simulink model "sampleModel1426_2_sub_sub_sub"  (R2023a)
settings: Solver=VariableStepAuto  StartTime=0.0  StopTime=10.0  RelTol=1e-3
libraries: hdlsllib x6, simulink x3
settings Model: Creator=user1  LastModifiedBy=user1
settings OptimizationCC: BlockReduction=off  ConditionallyExecuteInputs=off

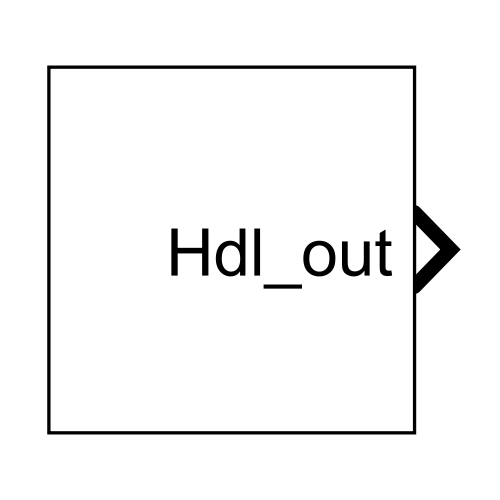
[thumbnail: Simulink's stored preview of the top-level diagram]
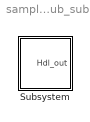
== system sampleModel1426_2_sub_sub_sub ==
  Subsystem : Subsystem

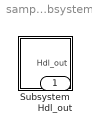
== system sampleModel1426_2_sub_sub_sub/Subsystem ==
  Subsystem : Subsystem
  Hdl_out : Outport  OutDataTypeStr=uint8

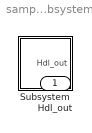
== system sampleModel1426_2_sub_sub_sub/Subsystem/Subsystem ==
  Subsystem : Subsystem
  Hdl_out : Outport  OutDataTypeStr=uint8

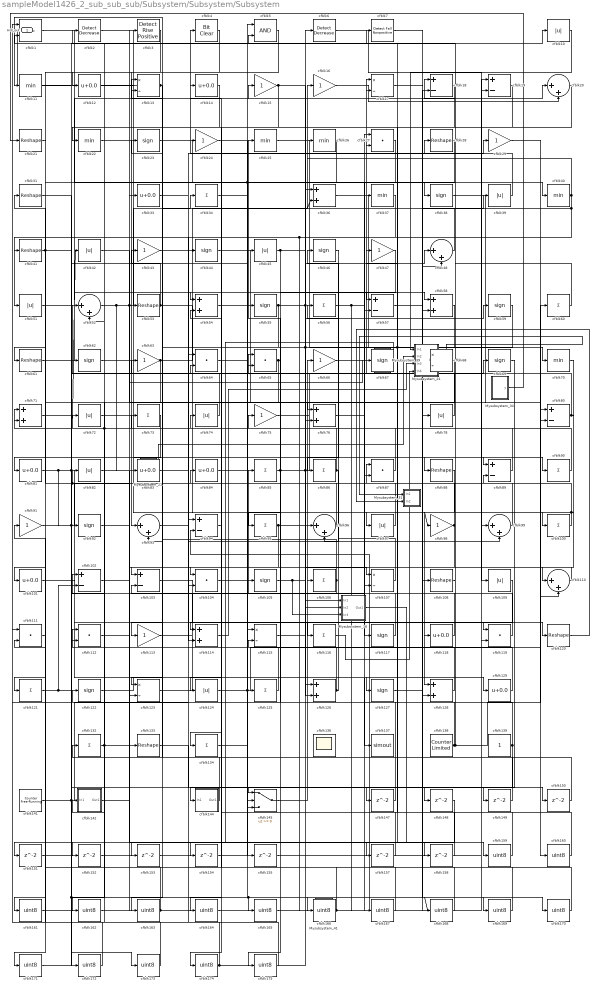
== system sampleModel1426_2_sub_sub_sub/Subsystem/Subsystem/Subsystem ==
  Mysubsystem_16 : Subsystem  TreatAsAtomicUnit=on  RTWFcnName=Mysubsystem_16
      settings: RTWFcnNameOpts=User specified  RTWFileNameOpts=Use function name
  Mysubsystem_21 : Subsystem  TreatAsAtomicUnit=on  RTWFcnName=Mysubsystem_21
      settings: RTWFcnNameOpts=User specified  RTWFileNameOpts=Use function name
  Mysubsystem_24 : Subsystem  TreatAsAtomicUnit=on  RTWFcnName=Mysubsystem_24
      settings: RTWFcnNameOpts=User specified  RTWFileNameOpts=Use function name
  Mysubsystem_31 : Subsystem  TreatAsAtomicUnit=on  RTWFcnName=Mysubsystem_31
      settings: RTWFcnNameOpts=User specified  RTWFileNameOpts=Use function name
  Mysubsystem_34 : Subsystem  TreatAsAtomicUnit=on  RTWFcnName=Mysubsystem_34
      settings: RTWFcnNameOpts=User specified  RTWFileNameOpts=Use function name
  Mysubsystem_39 : Subsystem  TreatAsAtomicUnit=on  RTWFcnName=Mysubsystem_39
      settings: RTWFcnNameOpts=User specified  RTWFileNameOpts=Use function name
  Mysubsystem_41 : Subsystem  TreatAsAtomicUnit=on  RTWFcnName=Mysubsystem_41
      settings: RTWFcnNameOpts=User specified  RTWFileNameOpts=Use function name
  cfblk1 : RelationalOperator  Operator=<=  OutDataTypeStr=boolean  InputSameDT=off
  cfblk{10,39,42,45,51,72,74,78,82,97,109,124} (12 alike) : Abs  OutDataTypeStr=uint8  SaturateOnIntegerOverflow=off
  cfblk{34,56,60,73,85..86,90,95,100,106,116,121,125,132,134} (15 alike) : Sum  Inputs=+  OutDataTypeStr=uint8
  cfblk{12,14,33,81,83..84,101,118,129} (9 alike) : Bias  Bias=0.0  SaturateOnIntegerOverflow=off
  cfblk{18..19,57,80,89,94,102..103} (8 alike) : Sum  Inputs=+-  OutDataTypeStr=uint8
  cfblk{27,64..65,87,104,111..112,119} (8 alike) : DotProduct  OutDataTypeStr=uint8
  cfblk{23,38,44,46,55,59,62,67,69,92,105,117,122,127} (14 alike) : Signum
  cfblk{13,17,68,107,115,123} (6 alike) : Product  Inputs=*/  OutDataTypeStr=uint8  RndMeth=Zero  SaturateOnIntegerOverflow=on
  cfblk{21,28,31,41,53,61,88,108,120,133} (10 alike) : Reshape
  cfblk{11,22,25..26,37,40,70} (7 alike) : MinMax  OutDataTypeStr=uint8
  cfblk{20,48,52,93,96,99,110} (7 alike) : Sum  Inputs=|++  OutDataTypeStr=uint8
  cfblk{15..16,24,29,43,47,63,66,75,91,98,113} (12 alike) : Gain  OutDataTypeStr=uint8
  cfblk{36,54,58,71,76,114,126,128} (8 alike) : Sum  OutDataTypeStr=uint8
  cfblk136 : Scope
      settings: Floating=on
  cfblk137 : ToWorkspace  VariableName=simout  SaveFormat=Timeseries  SampleTime=-1
  cfblk138 : hdlsllib/Sources/Counter Limited  uplimit=7  tsamp=-1
  cfblk139 : Constant  OutDataTypeStr=uint8  SampleTime=-1
  cfblk141 : hdlsllib/Sources/Counter Free-Running  NumBits=16  tsamp=-1
  cfblk142 : Subsystem
      settings: LibrarySourceBlock=|
      | hdlsllib/Ports &
      | Subsystems/Subsystem
  cfblk144 : Subsystem
      settings: LibrarySourceBlock=|
      | hdlsllib/Ports &
      | Subsystems/Subsystem
  cfblk145 : Switch  OutDataTypeStr=uint8  SaturateOnIntegerOverflow=off  InputSameDT=off
  cfblk{147..155,157..158} (11 alike) : Delay  SampleTime=1
  cfblk{159..175} (17 alike) : DataTypeConversion  OutDataTypeStr=uint8  SaturateOnIntegerOverflow=off  RndMeth=Floor
  cfblk2 : simulink/Logic and Bit Operations/Detect Decrease  vinit=0.0  OutDataTypeStr=uint8
      settings: LibrarySourceBlock=|
      | hdlsllib/Logic and Bit
      | Operations/Detect
      | Decrease
  cfblk3 : hdlsllib/Logic and Bit Operations/Detect Rise Positive  vinit=0  OutDataTypeStr=uint8
  cfblk4 : simulink/Logic and Bit Operations/Bit Clear  iBit=0
      settings: LibrarySourceBlock=|
      | hdlsllib/Logic and Bit
      | Operations/Bit Clear
  cfblk5 : Logic  AllPortsSameDT=off  OutDataTypeStr=boolean
  cfblk6 : simulink/Logic and Bit Operations/Detect Decrease  vinit=0.0  OutDataTypeStr=uint8
      settings: LibrarySourceBlock=|
      | hdlsllib/Logic and Bit
      | Operations/Detect
      | Decrease
  cfblk7 : hdlsllib/Logic and Bit Operations/Detect Fall Nonpositive  vinit=0  OutDataTypeStr=uint8
  Hdl_out : Outport  OutDataTypeStr=uint8
  wires:
  cfblk2/1 -> cfblk88/1
  cfblk48/1 -> cfblk11/1
  cfblk5/1 -> cfblk93/1
  cfblk54/1 -> cfblk25/1
  cfblk52/1 -> cfblk83/1, cfblk80/2, cfblk34/1
  cfblk64/1 -> cfblk166/1
  cfblk119/1 -> cfblk85/1
  cfblk117/1 -> cfblk66/1
  cfblk108/1 -> cfblk18/1
  cfblk53/1 -> cfblk43/1, cfblk97/1
  cfblk75/1 -> cfblk17/1
  cfblk33/1 -> cfblk29/1
  cfblk62/1 -> cfblk90/1
  cfblk61/1 -> cfblk15/1
  cfblk68/1 -> cfblk113/1
  cfblk101/1 -> cfblk120/1
  cfblk94/1 -> cfblk174/1
  cfblk1/1 -> cfblk38/1
  cfblk88/1 -> cfblk128/1
  cfblk56/1 -> cfblk167/1, cfblk117/1
  cfblk145/1 -> cfblk106/1
  cfblk58/1 -> cfblk157/1, cfblk123/1
  cfblk124/1 -> cfblk17/2, cfblk60/1
  cfblk6/1 -> cfblk99/1
  cfblk45/1 -> cfblk175/1, cfblk28/1
  cfblk110/1 -> cfblk104/1
  cfblk80/1 -> cfblk13/2, cfblk110/1
  cfblk38/1 -> cfblk110/2
  cfblk82/1 -> cfblk133/1
  cfblk122/1 -> cfblk127/1
  cfblk63/1 -> cfblk121/1, cfblk16/1
  cfblk107/1 -> cfblk75/1
  cfblk20/1 -> cfblk128/2
  cfblk72/1 -> cfblk118/1
  cfblk25/1 -> cfblk108/1
  cfblk74/1 -> cfblk63/1
  cfblk73/1 -> cfblk81/1
  cfblk12/1 -> cfblk40/1
  cfblk89/1 -> cfblk2/1, cfblk42/1
  cfblk36/1 -> cfblk70/1
  cfblk127/1 -> cfblk39/1
  cfblk141/1 -> cfblk44/1, cfblk173/1, cfblk168/1, cfblk165/1
  cfblk100/1 -> cfblk89/2, cfblk98/1
  cfblk85/1 -> cfblk65/1, cfblk59/1, cfblk69/1
  cfblk132/1 -> cfblk112/1, cfblk67/1
  cfblk86/1 -> cfblk96/2, cfblk71/1
  cfblk123/1 -> cfblk6/1
  cfblk103/1 -> cfblk116/1
  cfblk43/1 -> cfblk76/1
  cfblk144/1(Out1) -> cfblk132/1
  cfblk4/1 -> cfblk12/1
  cfblk129/1 -> cfblk115/2
  cfblk11/1 -> cfblk5/2
  cfblk118/1 -> cfblk87/1
  cfblk142/1(Out1) -> cfblk53/1
  cfblk22/1 -> cfblk57/1
  cfblk81/1 -> cfblk92/1, cfblk10/1, cfblk137/1
  cfblk44/1 -> cfblk109/1
  cfblk125/1 -> cfblk73/1
  cfblk83/1 -> cfblk99/2
  cfblk66/1 -> cfblk119/1
  cfblk90/1 -> cfblk23/1
  cfblk37/1 -> cfblk51/1
  cfblk21/1 -> cfblk61/1
  cfblk113/1 -> cfblk37/1
  cfblk39/1 -> cfblk4/1
  cfblk92/1 -> cfblk20/1
  cfblk93/1 -> cfblk27/2
  cfblk34/1 -> cfblk129/1
  cfblk51/1 -> cfblk54/1
  cfblk106/1 -> cfblk103/2, cfblk72/1
  cfblk26/1 -> cfblk114/1
  cfblk138/1 -> cfblk55/1, cfblk80/1, cfblk68/1
  cfblk121/1 -> cfblk102/2, cfblk105/1
  cfblk14/1 -> cfblk22/1
  cfblk19/1 -> cfblk163/1
  cfblk104/1 -> cfblk125/1
  cfblk139/1 -> cfblk52/2, cfblk144/1(In1)
  cfblk96/1 -> cfblk56/1, cfblk71/2, cfblk82/1
  cfblk46/1 -> cfblk86/1
  cfblk128/1 -> cfblk54/2
  cfblk41/1 -> cfblk145/3, cfblk101/1
  cfblk95/1 -> cfblk123/2, cfblk36/1
  cfblk115/1 -> cfblk48/1
  cfblk59/1 -> cfblk134/1, Mysubsystem_16/2(In2)
  cfblk16/1 -> cfblk20/2
  cfblk126/1 -> cfblk102/1, cfblk46/1
  cfblk70/1 -> cfblk100/1
  cfblk109/1 -> cfblk124/1
  cfblk87/1 -> cfblk74/1
  cfblk15/1 -> cfblk164/1, cfblk107/2
  cfblk55/1 -> cfblk103/1, cfblk58/1, Mysubsystem_16/1(In1)
  cfblk78/1 -> cfblk52/1
  cfblk105/1 -> cfblk107/1, Mysubsystem_16/3(In3)
  cfblk98/1 -> cfblk13/1, cfblk104/2
  cfblk28/1 -> cfblk57/2
  cfblk91/1 -> cfblk45/1, cfblk33/1
  cfblk60/1 -> cfblk1/2
  cfblk47/1 -> cfblk145/1
  cfblk23/1 -> cfblk126/2
  cfblk97/1 -> cfblk31/1
  cfblk27/1 -> cfblk65/2, cfblk41/1
  cfblk57/1 -> cfblk18/2
  cfblk40/1 -> cfblk26/1, cfblk36/2, cfblk114/2, Mysubsystem_41/1(In1)
  cfblk71/1 -> cfblk68/2
  cfblk67/1 -> cfblk47/1
  cfblk99/1 -> cfblk24/1
  cfblk65/1 -> cfblk152/1, cfblk95/1
  cfblk76/1 -> cfblk89/1
  cfblk18/1 -> cfblk147/1
  cfblk147/1 -> cfblk1/1
  cfblk133/1 -> cfblk148/1
  cfblk69/1 -> cfblk149/1
  cfblk149/1 -> cfblk93/2
  cfblk134/1 -> cfblk150/1
  cfblk150/1 -> cfblk126/1
  cfblk151/1 -> cfblk119/2
  cfblk152/1 -> cfblk145/2
  cfblk13/1 -> Hdl_out/1, cfblk153/1
  cfblk153/1 -> cfblk96/1
  cfblk154/1 -> cfblk48/2
  cfblk24/1 -> cfblk155/1
  cfblk155/1 -> cfblk27/1
  cfblk157/1 -> cfblk115/1
  cfblk102/1 -> cfblk158/1
  cfblk158/1 -> cfblk5/1
  cfblk7/1 -> cfblk159/1
  cfblk159/1 -> cfblk14/1
  cfblk29/1 -> cfblk160/1
  cfblk160/1 -> cfblk7/1
  cfblk3/1 -> cfblk161/1
  cfblk161/1 -> cfblk78/1
  cfblk148/1 -> cfblk162/1
  cfblk162/1 -> cfblk3/1
  cfblk163/1 -> cfblk87/2, cfblk112/2
  cfblk164/1 -> cfblk19/1
  cfblk165/1 -> cfblk19/2
  cfblk166/1 -> cfblk91/1, cfblk58/2
  cfblk167/1 -> cfblk64/1
  cfblk168/1 -> cfblk64/2
  cfblk84/1 -> cfblk169/1
  cfblk169/1 -> cfblk142/1(In1)
  cfblk17/1 -> cfblk170/1
  cfblk170/1 -> cfblk84/1
  cfblk111/1 -> cfblk171/1
  cfblk171/1 -> cfblk62/1
  cfblk31/1 -> cfblk172/1
  cfblk172/1 -> cfblk111/1
  cfblk173/1 -> cfblk111/2
  cfblk174/1 -> cfblk122/1, cfblk76/2
  cfblk175/1 -> cfblk94/1
  Mysubsystem_16/1(Out1) -> cfblk151/1
  cfblk112/1 -> Mysubsystem_21/1(In1)
  cfblk10/1 -> Mysubsystem_24/1(In1)
  Mysubsystem_21/1(Out1) -> Mysubsystem_24/2(In2)
  cfblk114/1 -> Mysubsystem_24/3(In3)
  cfblk116/1 -> Mysubsystem_24/4(In4)
  Mysubsystem_24/1(Out1) -> Mysubsystem_31/1(In1)
  cfblk120/1 -> Mysubsystem_31/2(In2)
  Mysubsystem_34/1(y) -> cfblk21/1
  cfblk42/1 -> Mysubsystem_39/1(In1)
  Mysubsystem_39/1(Out1) -> cfblk154/1
  Mysubsystem_41/1(Out1) -> cfblk94/2

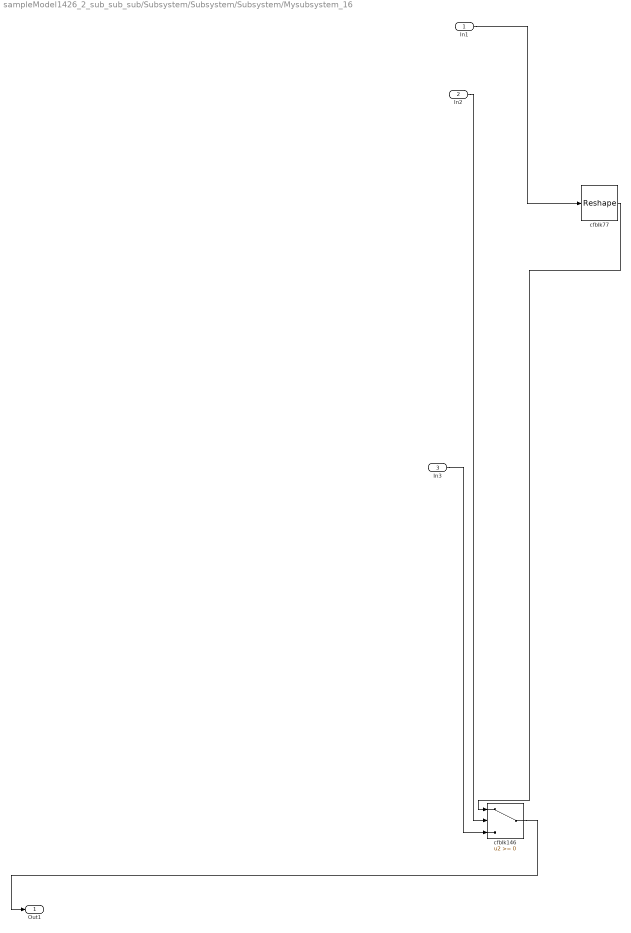
== system sampleModel1426_2_sub_sub_sub/Subsystem/Subsystem/Subsystem/Mysubsystem_16 ==
  In1 : Inport
  In2 : Inport  Port=2
  In3 : Inport  Port=3
  cfblk146 : Switch  SaturateOnIntegerOverflow=off  InputSameDT=off
  cfblk77 : Reshape
  Out1 : Outport
  wires:
  cfblk146/1 -> Out1/1
  In3/1 -> cfblk146/3
  In1/1 -> cfblk77/1
  In2/1 -> cfblk146/2
  cfblk77/1 -> cfblk146/1

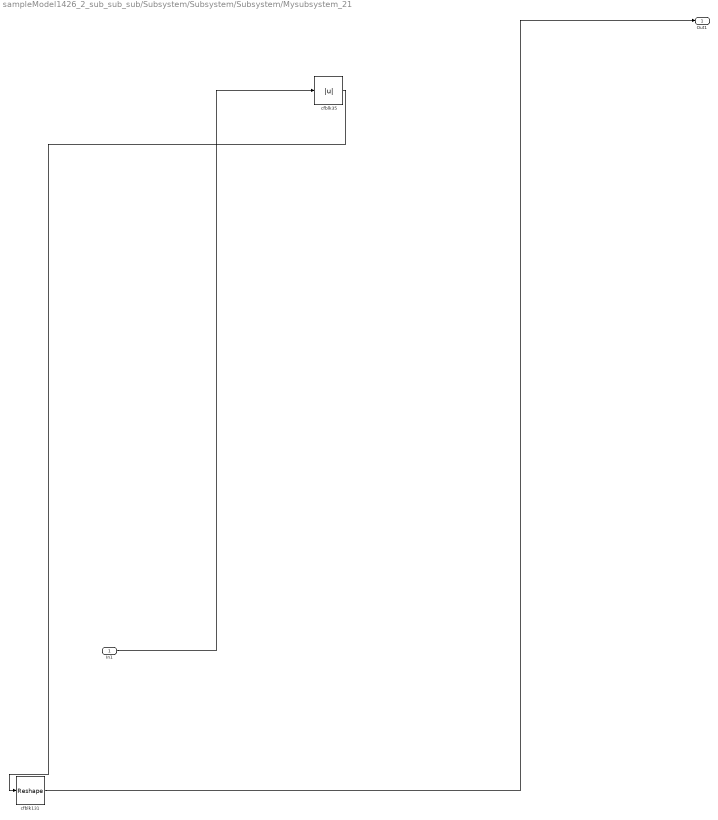
== system sampleModel1426_2_sub_sub_sub/Subsystem/Subsystem/Subsystem/Mysubsystem_21 ==
  In1 : Inport
  cfblk131 : Reshape
  cfblk35 : Abs  SaturateOnIntegerOverflow=off
  Out1 : Outport
  wires:
  In1/1 -> cfblk35/1
  cfblk35/1 -> cfblk131/1
  cfblk131/1 -> Out1/1

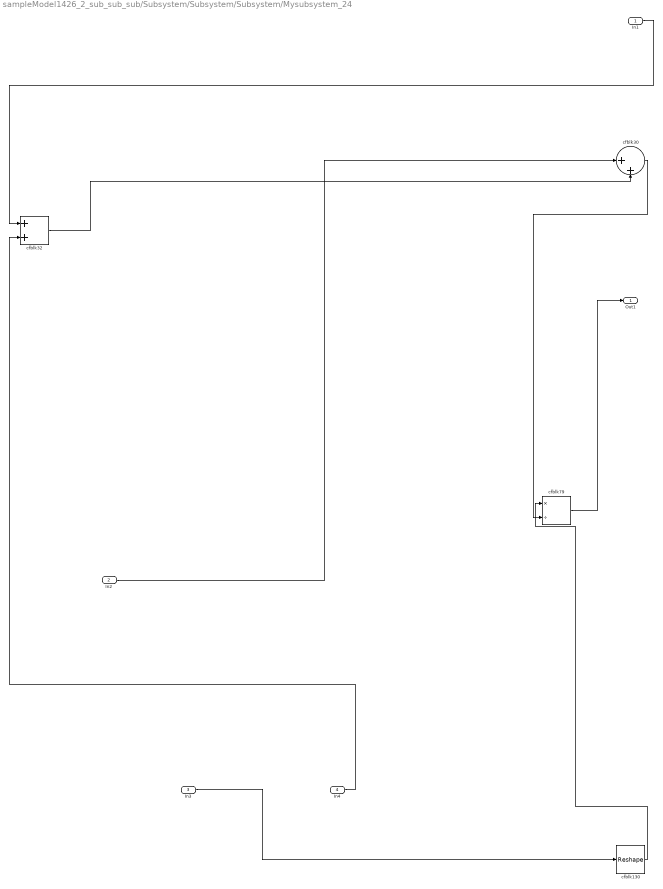
== system sampleModel1426_2_sub_sub_sub/Subsystem/Subsystem/Subsystem/Mysubsystem_24 ==
  In1 : Inport
  In2 : Inport  Port=2
  In3 : Inport  Port=3
  In4 : Inport  Port=4
  cfblk130 : Reshape
  cfblk30 : Sum  Inputs=|++
  cfblk32 : Sum
  cfblk79 : Product  Inputs=*/  RndMeth=Zero  SaturateOnIntegerOverflow=on
  Out1 : Outport
  wires:
  In2/1 -> cfblk30/1
  cfblk79/1 -> Out1/1
  In3/1 -> cfblk130/1
  cfblk32/1 -> cfblk30/2
  In1/1 -> cfblk32/1
  cfblk130/1 -> cfblk79/1
  cfblk30/1 -> cfblk79/2
  In4/1 -> cfblk32/2

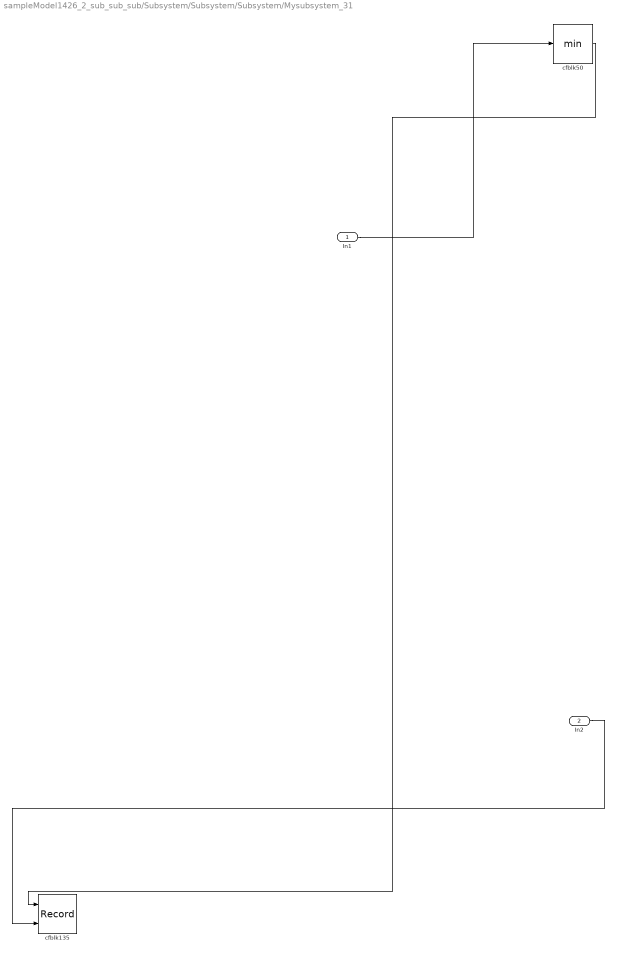
== system sampleModel1426_2_sub_sub_sub/Subsystem/Subsystem/Subsystem/Mysubsystem_31 ==
  In1 : Inport
  In2 : Inport  Port=2
  cfblk135 : Record  FileSettingsInternal="{\"entries\":[{\"content\":{\"excelSettings\":{\"content\":{},\"type\":\"Streamout.ExcelSettings\"}},\"type\":\"Streamout.FileSettingStorage\",\"uuid\":\"\"}],\"packageUris\":[\"http:\\/\\/schema.mathworks.com\\/mf0\\/streamout_blocks\\/R2020a\"],\"version\":\"1.0\"}"  Layout=[1 1]  SignalsInternal="{\"entries\":[{\"content\":{},\"type\":\"RecordBlkView.InputSignals\",\"uuid\":\"\"}],\"packageUris\":[\"http:\\/\\/schema.mathworks.com\\/mf0\\/streamout_blocks\\/R2020a\"],\"version\":\"1.0\"}"  VisualizationBindings="{\"xyplotplugin\":{\"info\":[{\"series\":[],\"subplotID\":1}]}}"  CompatibilityTag=XY  st=-1
  cfblk50 : MinMax
  wires:
  In2/1 -> cfblk135/2
  In1/1 -> cfblk50/1
  cfblk50/1 -> cfblk135/1

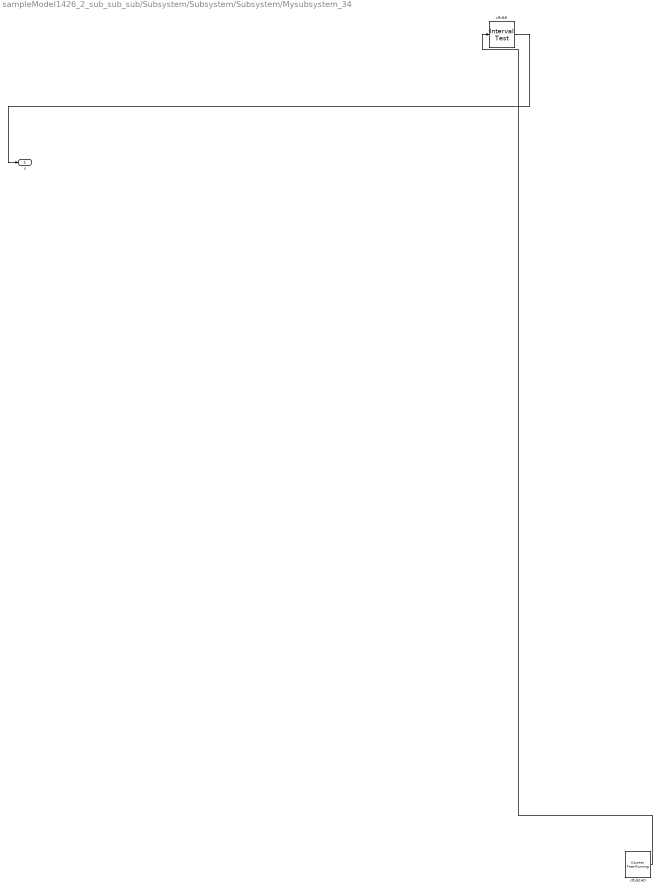
== system sampleModel1426_2_sub_sub_sub/Subsystem/Subsystem/Subsystem/Mysubsystem_34 ==
  cfblk140 : hdlsllib/Sources/Counter Free-Running  NumBits=16  tsamp=-1
  cfblk8 : hdlsllib/Logic and Bit Operations/Interval Test  IntervalClosedRight=on  uplimit=0.5  IntervalClosedLeft=on  lowlimit=-0.5  OutDataTypeStr=boolean
  y : Outport
  wires:
  cfblk8/1 -> y/1
  cfblk140/1 -> cfblk8/1

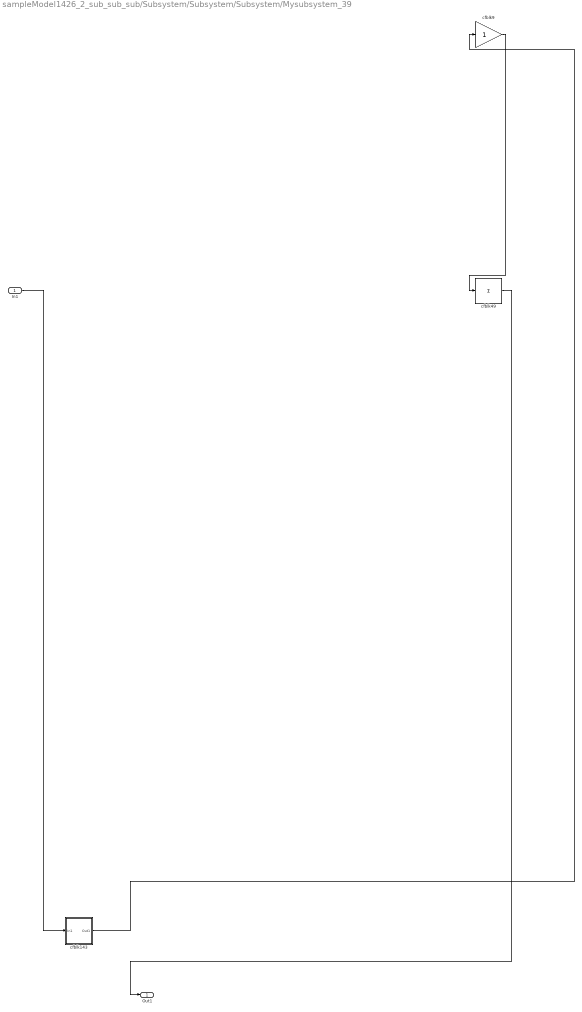
== system sampleModel1426_2_sub_sub_sub/Subsystem/Subsystem/Subsystem/Mysubsystem_39 ==
  In1 : Inport
  cfblk143 : Subsystem
      settings: LibrarySourceBlock=|
      | hdlsllib/Ports &
      | Subsystems/Subsystem
  cfblk49 : Sum  Inputs=+
  cfblk9 : Gain
  Out1 : Outport
  wires:
  cfblk143/1(Out1) -> cfblk9/1
  cfblk49/1 -> Out1/1
  cfblk9/1 -> cfblk49/1
  In1/1 -> cfblk143/1(In1)

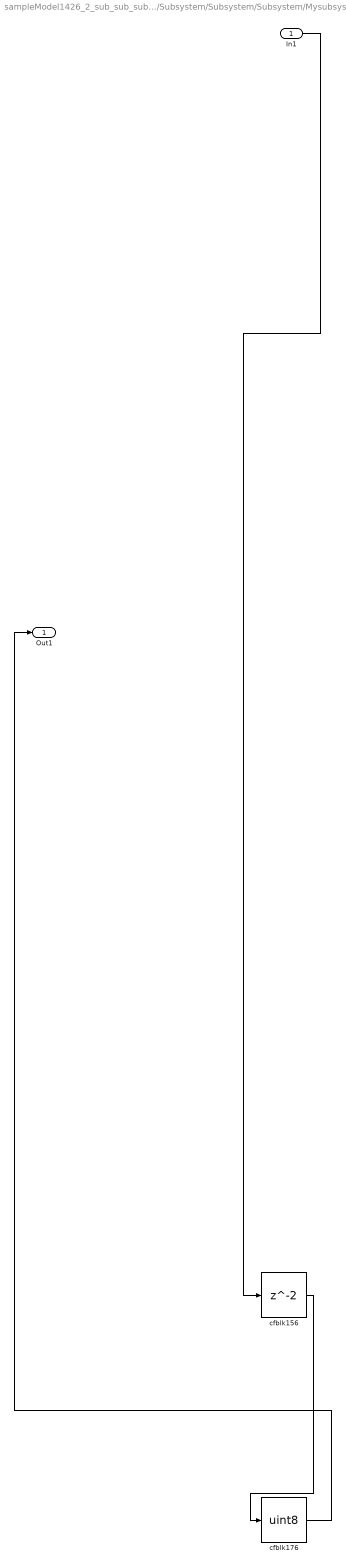
== system sampleModel1426_2_sub_sub_sub/Subsystem/Subsystem/Subsystem/Mysubsystem_41 ==
  In1 : Inport
  cfblk156 : Delay  SampleTime=1
  cfblk176 : DataTypeConversion  OutDataTypeStr=uint8  SaturateOnIntegerOverflow=off  RndMeth=Floor
  Out1 : Outport
  wires:
  In1/1 -> cfblk156/1
  cfblk156/1 -> cfblk176/1
  cfblk176/1 -> Out1/1

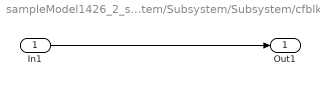
== system sampleModel1426_2_sub_sub_sub/Subsystem/Subsystem/Subsystem/cfblk142 ==
  In1 : Inport
  Out1 : Outport
  wires:
  In1/1 -> Out1/1

== system sampleModel1426_2_sub_sub_sub/Subsystem/Subsystem/Subsystem/cfblk144 ==
  In1 : Inport
  Out1 : Outport
  wires:
  In1/1 -> Out1/1

== system sampleModel1426_2_sub_sub_sub/Subsystem/Subsystem/Subsystem/Mysubsystem_39/cfblk143 ==
  In1 : Inport
  Out1 : Outport
  wires:
  In1/1 -> Out1/1
